simulink model "Model1F"  (R2014b)
settings: Solver=ode23tb  StartTime=0.0  StopTime=0.1  MaxStep=10e-6  RelTol=1e-3
values from neighbouring files (symbols this model uses):
  D = 50    [Parametri.m]
  R = 10    [Parametri.m]
  T = 1/f    (= 0.02)    [Parametri.m]
  Vg = 450    [Parametri.m]
undefined symbols (not defined in the file or in its folder): L
libraries: powerlib x10
settings Model: Creator=Zorana  LastModifiedBy=Zorana

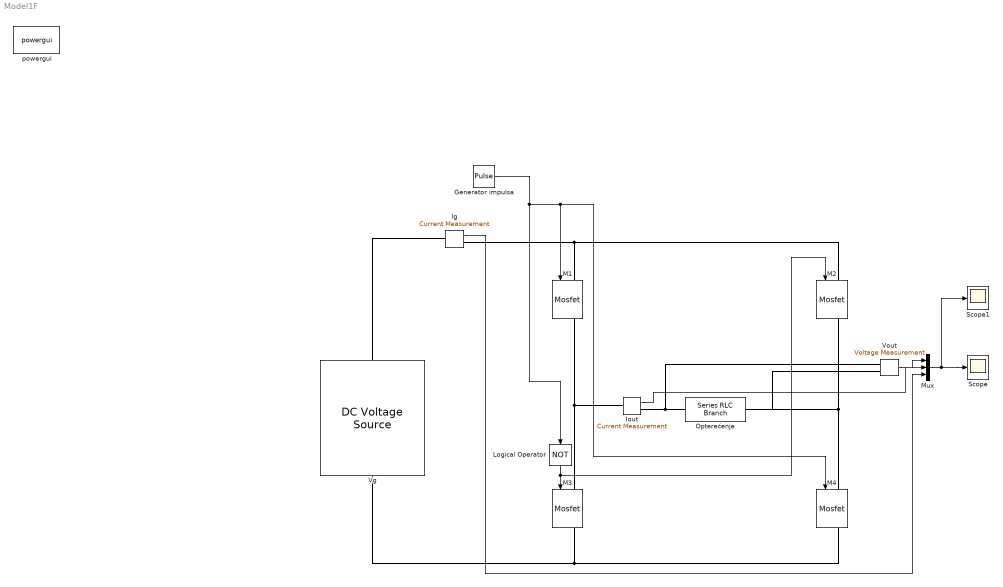
== system Model1F ==
  Generator impulsa : DiscretePulseGenerator  PulseType=Time based  Period=T  PulseWidth=D
  Ig : powerlib/Measurements/Current Measurement  PhasorSimulation=off  OutputType=Complex  PSBequivalent=0
  Iout : powerlib/Measurements/Current Measurement  PhasorSimulation=off  OutputType=Complex  PSBequivalent=0
  Logical Operator : Logic  Operator=NOT  IconShape=distinctive  AllPortsSameDT=off  OutDataTypeStr=boolean
  M{1..4} (4 alike) : powerlib/Power Electronics/Mosfet  Ron=1e-6  Lon=0  Rd=1e-6  Vfd=0  IC=0  Rs=1e5  Cs=inf  Measurements=on
  Mux : Mux  Inputs=3
  Opterećenje : powerlib/Elements/Series RLC Branch  LConnTagsString=__new0  RConnTagsString=__new0  BranchType=RL  Resistance=R  Inductance=L  SetiL0=off  InitialCurrent=0  Capacitance=1e-6  Setx0=off  InitialVoltage=0  Measurements=None
  Scope : Scope
  Scope1 : Scope
  Vg : powerlib/Electrical Sources/DC Voltage Source  Amplitude=Vg  Measurements=None
  Vout : powerlib/Measurements/Voltage Measurement  PhasorSimulation=off  OutputType=Complex  PSBequivalent=0
  powergui : powerlib/powergui  Priority=1  SimulationMode=Continuous  SolverType=Tustin/Backward Euler (TBE)  SampleTime=50e-6  frequency=60  SPID=off  DisableSnubberDevices=off  DisableRonSwitches=off  DisableVfSwitches=off  SwTol=0  DisplayEquations=off  Interpol=off  methode=off  Ts=100  frequencyindice=0  Pbase=100e6  ErrMax=1e-4  Iterations=50  UnitsV=kV  UnitsW=MW  FunctionMessages=off  echomessages=off  HookPort=off  EnableUseOfTLC=off  x0status=blocks  RestoreLinks=warning  ResistiveCurrentMeasurement=off  Frange=[0:2:500]  Ylog=off  Xlog=on  ShowGrid=off  save=off  variable=ZData  structure=0  ZoomFFT=off  StartTime=0.0  cycles=1  DisplayStyle=1  fundamental=60  FreqAxis=off  MaxFrequency=1000  frequencyindicesteady=1  RmsSteady=1  display=off
  wires:
  Vout/1 -> Mux/1
  Iout/1 -> Mux/2
  Mux/1 -> Scope1/1, Scope/1
  Generator impulsa/1 -> Logical Operator/1, M4/1, M1/1
  Logical Operator/1 -> M2/1, M3/1
  Ig/1 -> Mux/3
  connections:
  M1/RConn1 -- Iout/LConn1 -- M3/LConn1
  M3/RConn1 -- M4/RConn1 -- Vg/LConn1
  M2/RConn1 -- Vout/LConn2 -- Opterećenje/RConn1 -- M4/LConn1
  M1/LConn1 -- Ig/RConn1 -- M2/LConn1
  Iout/RConn1 -- Vout/LConn1 -- Opterećenje/LConn1
  Vg/RConn1 -- Ig/LConn1
